simulink model "handsteuer_Joystick"  (R2017a)
settings: Solver=ode4  StartTime=0.0  StopTime=10  FixedStep=0.01  RelTol=1e-3  EnableMultiTasking=on
undefined symbols (not defined in the file or in its folder): Joystick, National_Instruments, PCIe, Standard_Devices
libraries: sldrtlib x3, cstblocks x1
CloseFcn:
  | rtwprivate ssgencode ModelCloseRequest handsteuer_Joystick
settings Model: SimulationMode=external  ExtModeTrigDuration=1000000  Creator=Praktikum  LastModifiedBy=prt01
settings DataIOCC: LimitDataPoints=on  SaveFormat=Array  SignalLoggingSaveFormat=ModelDataLogs
settings OptimizationCC: ExpressionDepthLimit=2147483647  InitFltsAndDblsToZero=on
settings DebuggingCC: SaveWithParameterizedLinksMsg=none  UnderspecifiedInitializationDetection=Classic  MergeDetectMultiDrivingBlocksExec=none  SignalResolutionControl=TryResolveAllWithWarning  SolverPrmCheckMsg=warning  MultiTaskDSMMsg=warning  MultiTaskCondExecSysMsg=none  FcnCallInpInsideContextMsg=warning  StateNameClashWarn=warning  SFUnexpectedBacktrackingDiag=warning  SFNoUnconditionalDefaultTransitionDiag=warning  SFExecutionAtInitializationDiag=none
settings ModelReferenceCC: PropagateSignalLabelsOutOfModel=off
settings RTWCC: SystemTargetFile=sldrt.tlc  TemplateMakefile=sldrt.tmf  Description=Simulink Desktop Real-Time  RTWCompilerOptimization=on
settings CodeAppCC: MaxIdLength=95
settings SimulinkDesktopRealTimeCC: TargetFcnLib=ansi_tfl_tmw.mat  TargetPreCompLibLocation=C:\Program Files\MATLAB\R2017a\toolbox\sldrt\lib\win64  TargetLangStandard=C89/C90 (ANSI)  ModelReferenceCompliant=off  CompOptLevelCompliant=off  SupportVariableSizeSignals=off
settings ConfigComp: CovMetricSettings=dw  CovHtmlReporting=on  CovSaveCumulativeToWorkspaceVar=on  CovSaveSingleToWorkspaceVar=on  CovExternalEMLEnable=off

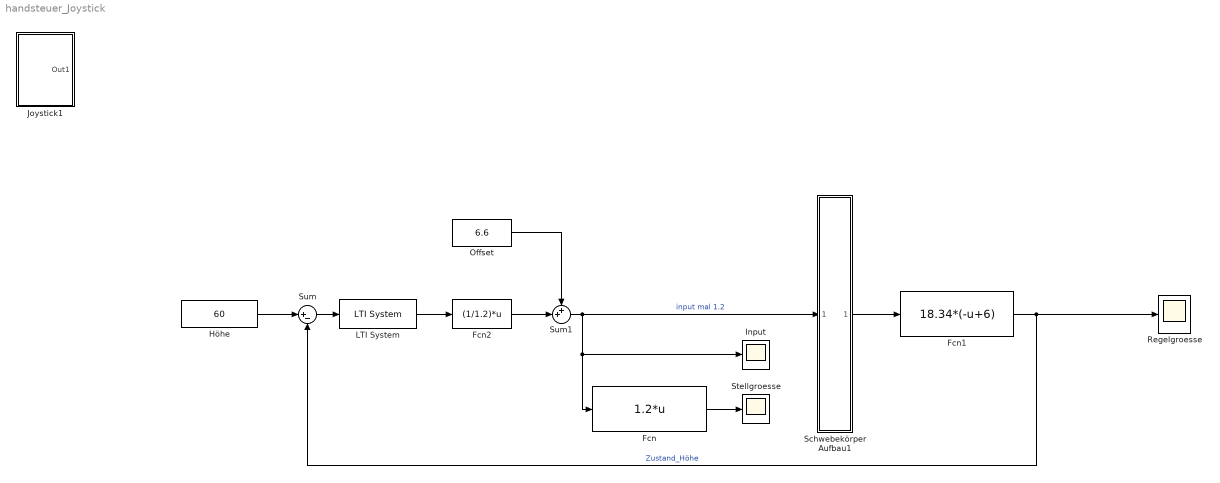
== system handsteuer_Joystick ==
  Fcn : Fcn  Expr=1.2*u
  Fcn1 : Fcn  Expr=18.34*(-u+6)
  Fcn2 : Fcn  Expr=(1/1.2)*u
  Höhe : Constant  Value=60
  Input : Scope
  Joystick1 : Subsystem
      mask Display: image(imread('Joystick.bmp'))
  LTI System : cstblocks/LTI System  sys=C  IC=[]
  "Offset " : Constant  Value=6.6
  Regelgroesse : Scope
  Schwebekörper Aufbau1 : Subsystem
      mask Display: image(imread('SKAufbauSkizze1.jpg'))
  Stellgroesse : Scope
  Sum : Sum  Inputs=|+-
  Sum1 : Sum  Inputs=++|
  wires:
  Fcn/1 -> Stellgroesse/1
  Schwebekörper Aufbau1/1(yAD) -> Fcn1/1
  Fcn1/1 -> Sum/2, Regelgroesse/1  "Zustand_Höhe"
  Sum1/1 -> Fcn/1, Input/1, Schwebekörper Aufbau1/1(uDA)  "input mal 1.2"
  Höhe/1 -> Sum/1
  LTI System/1 -> Fcn2/1
  "Offset "/1 -> Sum1/1
  Sum/1 -> LTI System/1
  Fcn2/1 -> Sum1/2

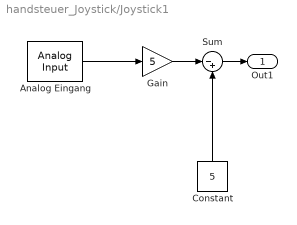
== system handsteuer_Joystick/Joystick1 ==
  Analog Eingang : sldrtlib/Analog Input  SampleTime=0.01  MaxMissedTicks=10  ShowMissedTicks=off  YieldWhenWaiting=off  DrvName=Standard_Devices/Joystick  DrvAddress=1  DrvOptions=zeros(1,0)  Channels=2  RangeMode=1  VoltRange=1  DataType=1
      settings: AttributesFormatString=Standard Devices\nJoystick [1h]  SourceProductName=Simulink Desktop Real-Time
  Constant : Constant  Value=5
  Gain : Gain  Gain=5
  Sum : Sum  Inputs=|-+
  Out1 : Outport
  wires:
  Sum/1 -> Out1/1
  Constant/1 -> Sum/2
  Gain/1 -> Sum/1
  Analog Eingang/1 -> Gain/1

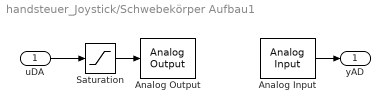
== system handsteuer_Joystick/Schwebekörper Aufbau1 ==
  uDA : Inport
  Analog Input : sldrtlib/Analog Input  SampleTime=0.01  MaxMissedTicks=10  ShowMissedTicks=off  YieldWhenWaiting=off  DrvName=National_Instruments/PCIe-6321  DrvAddress=4294967295  DrvOptions=[0 0 0 0 0 0 0]  Channels=1  RangeMode=1  VoltRange=1  DataType=1
      settings: AttributesFormatString=National Instruments\nPCIe-6321 [auto]  SourceProductName=Simulink Desktop Real-Time
  Analog Output : sldrtlib/Analog Output  SampleTime=0.01  MaxMissedTicks=10  ShowMissedTicks=off  YieldWhenWaiting=off  DrvName=National_Instruments/PCIe-6321  DrvAddress=4294967295  DrvOptions=[0 0 0 0 0 0 0]  Channels=1  RangeMode=1  VoltRange=1  InitialValue=0  FinalValue=0
      settings: AttributesFormatString=National Instruments\nPCIe-6321 [auto]  SourceProductName=Simulink Desktop Real-Time
  Saturation : Saturate  UpperLimit=10  LowerLimit=0
  yAD : Outport
  wires:
  Analog Input/1 -> yAD/1
  uDA/1 -> Saturation/1
  Saturation/1 -> Analog Output/1
